simulink model "HW_4_Q2"  (R2023b)
settings: Solver=VariableStepAuto  StartTime=0.0  StopTime=20  RelTol=1e-3
undefined symbols (not defined in the file): A, B, Cc, Dd, fnew, gx, H, K, Ov, Ox, oy, P, Q, ref, x0, Y, yc, yx
libraries: simulink x1
settings Model: Creator=mani8618  LastModifiedBy=Deven
settings DebuggingCC: UnconnectedInputMsg=warning  UnconnectedOutputMsg=warning  UnconnectedLineMsg=warning
settings ModelReferenceCC: EnableRefExpFcnMdlSchedulingChecks=on
settings RTWCC: DLArmComputeVersion=19.05

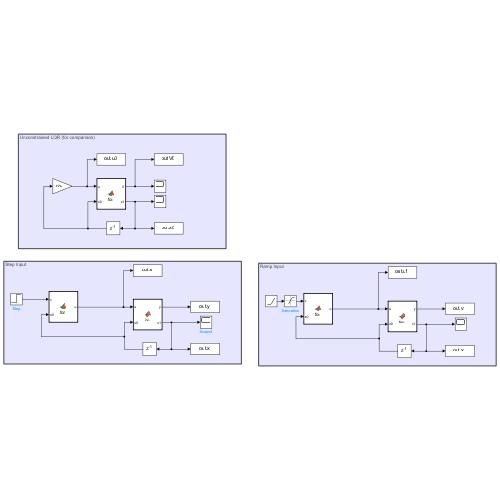
[thumbnail: Simulink's stored preview of the top-level diagram]
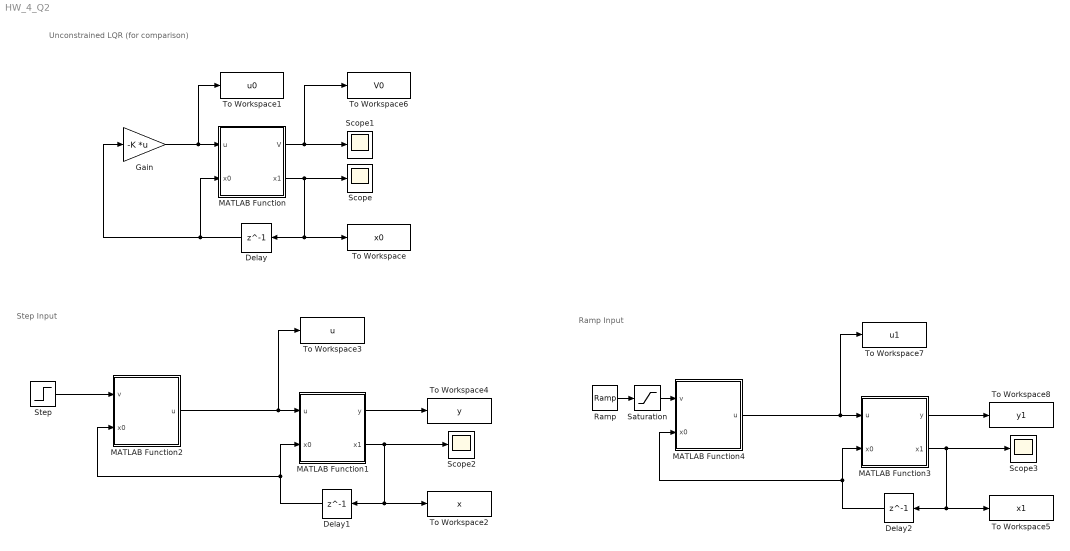
== system HW_4_Q2 ==
  note: Step Input
  note: Unconstrained LQR (for comparison)
  note: Ramp Input
  Delay : Delay  DelayLength=1  InitialCondition=x0  SampleTime=.1
  Delay1 : Delay  DelayLength=1  InitialCondition=x0  SampleTime=.1
  Delay2 : Delay  DelayLength=1  InitialCondition=x0  SampleTime=.1
  Gain : Gain  Gain=-K  Multiplication=Matrix(K*u)
  MATLAB Function : MATLAB Function  TreatAsAtomicUnit=on
  MATLAB Function1 : MATLAB Function  TreatAsAtomicUnit=on
  MATLAB Function2 : MATLAB Function  TreatAsAtomicUnit=on
  MATLAB Function3 : MATLAB Function  TreatAsAtomicUnit=on
  MATLAB Function4 : MATLAB Function  TreatAsAtomicUnit=on
  Ramp : simulink/Sources/Ramp  slope=10  start=0  InitialOutput=[0;0]
  Saturation : Saturate
  Scope{,1..3} (4 alike) : Scope
  Step : Step  After=ref  SampleTime=0
  To Workspace : ToWorkspace  VariableName=x0  SampleTime=-1
  To Workspace1 : ToWorkspace  VariableName=u0  SampleTime=-1
  To Workspace2 : ToWorkspace  VariableName=x  SampleTime=-1
  To Workspace3 : ToWorkspace  VariableName=u  SampleTime=-1
  To Workspace4 : ToWorkspace  VariableName=y  SampleTime=-1
  To Workspace5 : ToWorkspace  VariableName=x1  SampleTime=-1
  To Workspace6 : ToWorkspace  VariableName=V0  SampleTime=-1
  To Workspace7 : ToWorkspace  VariableName=u1  SampleTime=-1
  To Workspace8 : ToWorkspace  VariableName=y1  SampleTime=-1
  wires:
  MATLAB Function2/1(u) -> To Workspace3/1, MATLAB Function1/1(u)
  MATLAB Function/2(x1) -> Delay/1, To Workspace/1, Scope/1
  MATLAB Function/1(V) -> To Workspace6/1, Scope1/1
  Step/1 -> MATLAB Function2/1(v)
  Delay1/1 -> MATLAB Function1/2(x0), MATLAB Function2/2(x0)
  Delay/1 -> Gain/1, MATLAB Function/2(x0)
  MATLAB Function1/2(x1) -> Scope2/1, Delay1/1, To Workspace2/1
  MATLAB Function1/1(y) -> To Workspace4/1
  Gain/1 -> To Workspace1/1, MATLAB Function/1(u)
  MATLAB Function3/1(y) -> To Workspace8/1
  MATLAB Function3/2(x1) -> To Workspace5/1, Delay2/1, Scope3/1
  Delay2/1 -> MATLAB Function4/2(x0), MATLAB Function3/2(x0)
  Ramp/1 -> Saturation/1
  MATLAB Function4/1(u) -> MATLAB Function3/1(u), To Workspace7/1
  Saturation/1 -> MATLAB Function4/1(v)

== matlab function HW_4_Q2/MATLAB Function1 ==
  data: y output; u input; x1 output; x0 input; A parameter; B parameter; Cc parameter; Dd parameter
function [y,x1]   = fcn(u,x0,A,B,Cc, Dd)

x1 = A*x0+B*u;
y = Cc*x0+Dd*u;

end

== matlab function HW_4_Q2/MATLAB Function ==
  data: V output; u input; x1 output; x0 input; A parameter; B parameter; P parameter
function [V,x1] = fcn(u,x0,A,B,P)

x1 = A*x0+B*u;

V = x0'*P*x0;

end

== matlab function HW_4_Q2/MATLAB Function2 ==
  data: H parameter; u output; E parameter; gx parameter; Q parameter; Y parameter; yx parameter; yc parameter; Ox parameter; Ov parameter; oy parameter; fnew parameter; v input; x0 input
function u   = fcn(H,E,gx,Q,Y,yx,yc,Ox,Ov,oy, fnew, v, x0)
coder.extrinsic('quadprog');
coder.extrinsic('optimoptions');

% z = f;
z = -fnew*v;
z = quadprog(H,-fnew*v,[Y;Ox],[yc+yx*x0;oy-Ov*v],E,gx*x0,[],[],[],optimoptions('quadprog','Display','none'));
% z = quadprog(H,-fnew*v,Y,yc+yx*x0,E,gx*x0,[],[],[],optimoptions('quadprog','Display','none'));

% V = x0'*Q*x0+z'*H*z+f'*z;
u = z(1:2);
% u = z(1);

end

== matlab function HW_4_Q2/MATLAB Function3 ==
  data: y output; u input; x1 output; x0 input; A parameter; B parameter; Cc parameter; Dd parameter
function [y,x1]   = fcn(u,x0,A,B,Cc, Dd)

x1 = A*x0+B*u;
y = Cc*x0+Dd*u;

end

== matlab function HW_4_Q2/MATLAB Function4 ==
  data: H parameter; u output; E parameter; gx parameter; Q parameter; Y parameter; yx parameter; yc parameter; Ox parameter; Ov parameter; oy parameter; fnew parameter; v input; x0 input
function u   = fcn(H,E,gx,Q,Y,yx,yc,Ox,Ov,oy, fnew, v, x0)
coder.extrinsic('quadprog');
coder.extrinsic('optimoptions');

if v(1) > 5
    v(1) = 5;
end

v(2) = 0;
z = -fnew*v;
z = quadprog(H,-fnew*v,[Y;Ox],[yc+yx*x0;oy-Ov*v],E,gx*x0,[],[],[],optimoptions('quadprog','Display','none'));

u = z(1:2);

end
